simulink model "BPSK_Modem_v1_BMT_012314"  (R2013a)
settings: Solver=ode3  SolverMode=SingleTasking  StartTime=0.0  StopTime=10e3/2400  FixedStep=1/480e3  RelTol=1e-3
values from neighbouring files (symbols this model uses):
  Ki = 2.55    [Costas_Loop_Control_Design.m]
  Ko = ((r*s)/2)^2*H0^2    (= 0.015625)    [Costas_Loop_Control_Design.m]
  Kp = 4.41    [Costas_Loop_Control_Design.m]
  Kv = 2*pi*100    (= 628.318530718)    [Costas_Loop_Control_Design.m]
undefined symbols (not defined in the file or in its folder): DiscIntNeverNeededParam
libraries: commsynccomp2 x3, simulink x3, dspsigops x3, commutil2 x1, commchan3 x1, commrandsrc2 x1, commsink2 x1
settings Model: Creator=tibbs2010  LastModifiedBy=tibbs2010
settings DataIOCC: SignalLoggingSaveFormat=ModelDataLogs
settings DebuggingCC: MultiTaskDSMMsg=warning  MultiTaskCondExecSysMsg=none  StrictBusMsg=None
settings RTWCC: IncludeERTFirstTime=on

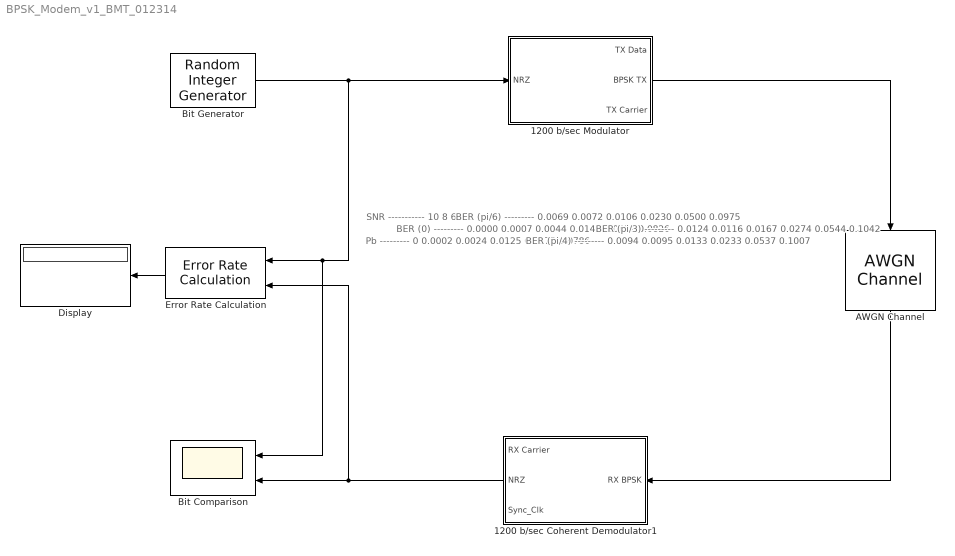
== system BPSK_Modem_v1_BMT_012314 ==
  note: BER (0)
      | ---------
      | 0.0000
      | 0.0007
      | 0.0044
      | 0.0144
      | 0.0432
      | 0.0826
  note: SNR
      | -----------
      |    10
      |      8
      |      6
      |      4
      |      2
      |      0
  note: Pb
      | ---------
      | 0
      | 0.0002
      | 0.0024
      | 0.0125
      | 0.0375
      | 0.0786
  note: BER (pi/6)
      | ---------
      | 0.0069
      | 0.0072
      | 0.0106
      | 0.0230
      | 0.0500
      | 0.0975
  note: BER (pi/4)
      | ---------
      | 0.0094
      | 0.0095
      | 0.0133
      | 0.0233
      | 0.0537
      | 0.1007
  note: BER (pi/3)
      | ---------
      | 0.0124
      | 0.0116
      | 0.0167
      | 0.0274
      | 0.0544
      | 0.1042
  1200 b/sec Modulator : Subsystem
  1200 b/sec Coherent Demodulator1 : Subsystem
  AWGN Channel : commchan3/AWGN Channel  InputProcessing=Columns as channels (frame based)  seed=randseed  noiseMode="Signal to noise ratio  (Eb/No)"  EbNodB=0  EsNodB=10  SNRdB=10  bitsPerSym=1  Ps=12.5  Tsym=1/2400  variance=1
  Bit Comparison : Scope  NumInputPorts=2
      settings: TimeRange=0.008608695652173926  YMin=-0.5~-0.5  YMax=1.5~1.5
  Bit Generator : commrandsrc2/Random Integer Generator  mul=2  seed=randseed  Ts=1/2400  frameBased=off  sampPerFrame=1  orient=off  outDataType=double
  Display : Display
  Error Rate Calculation : commsink2/Error Rate Calculation  N=3  st_delay=0  cp_mode=Entire frame  subframe=[]  PMode=Port  WsName=grayBER  RsMode2=off  stop=off  numErr=1072  maxBits=10e3
  wires:
  Error Rate Calculation/1 -> Display/1
  AWGN Channel/1 -> 1200 b/sec Coherent Demodulator1/1(RX BPSK)
  1200 b/sec Coherent Demodulator1/2(NRZ) -> Error Rate Calculation/2, Bit Comparison/2
  1200 b/sec Modulator/2(BPSK TX) -> AWGN Channel/1
  Bit Generator/1 -> Bit Comparison/1, Error Rate Calculation/1, 1200 b/sec Modulator/1(NRZ)

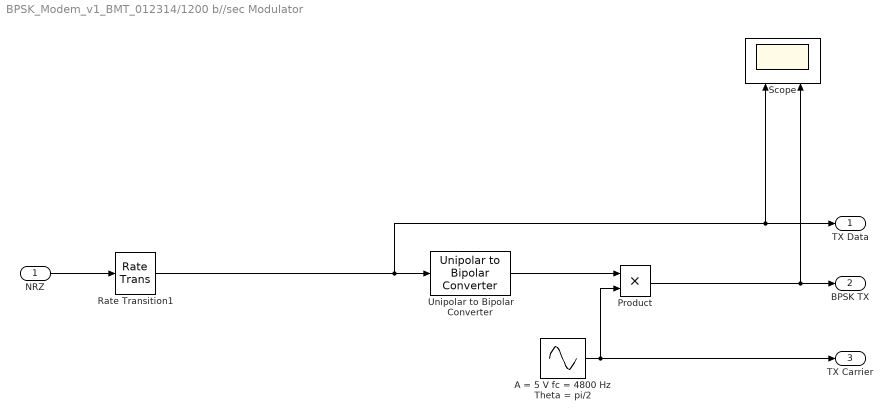
== system BPSK_Modem_v1_BMT_012314/1200 b//sec Modulator ==
  NRZ : Inport
  A = 5 V fc = 4800 Hz Theta = pi/2 : Sin  Amplitude=5  Frequency=2*pi*4800  Phase=pi/2  SampleTime=1/480e3
  Product : Product
  Rate Transition1 : RateTransition  OutPortSampleTime=1/480e3
  Scope : Scope  NumInputPorts=2
      settings: TimeRange=0.06  YMin=-0.5~-0.5  YMax=1.5~1.5  SaveName=ScopeData2
  Unipolar to Bipolar Converter : commutil2/Unipolar to Bipolar Converter  M=2  polarity=Positive  dataType=Inherit via internal rule
  TX Data : Outport
  BPSK TX : Outport  Port=2
  TX Carrier : Outport  Port=3
  wires:
  Rate Transition1/1 -> TX Data/1, Scope/1, Unipolar to Bipolar Converter/1
  Unipolar to Bipolar Converter/1 -> Product/1
  A = 5 V fc = 4800 Hz Theta = pi/2/1 -> TX Carrier/1, Product/2
  NRZ/1 -> Rate Transition1/1
  Product/1 -> Scope/2, BPSK TX/1

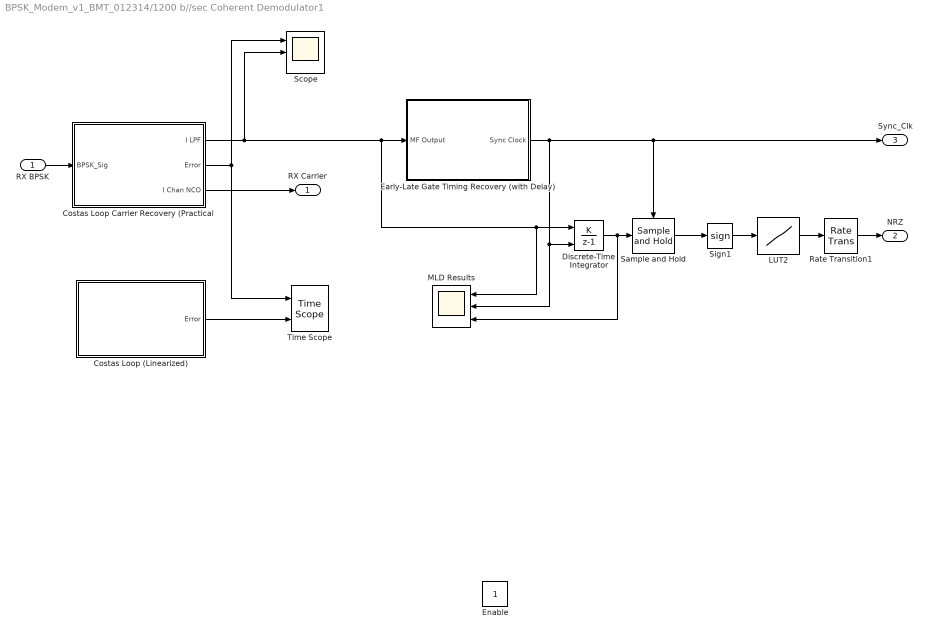
== system BPSK_Modem_v1_BMT_012314/1200 b//sec Coherent Demodulator1 ==
  RX BPSK : Inport
  Costas Loop Carrier Recovery (Practical : Subsystem
  Costas Loop (Linearized) : Subsystem
  Discrete-Time Integrator : DiscreteIntegrator  IntegratorMethod=Accumulation: Forward Euler  ExternalReset=rising  SampleTime=1/480e3  ICPrevOutput=DiscIntNeverNeededParam  ICPrevScaledInput=DiscIntNeverNeededParam
  Early-Late Gate Timing Recovery (with Delay) : Subsystem
  Enable : Constant
  LUT2 : Lookup_n-D  NumberOfTableDimensions=1  BreakpointsForDimension1=[-1 0 1]  Table=[0 0 1]  RndMeth=Simplest  InputSameDT=on
  MLD Results : Scope  NumInputPorts=3
      settings: TimeRange=0.01093750000000002  YMin=-0.5~-0.5~-5  YMax=1.5~1.5~5  SaveName=ScopeData4
  Rate Transition1 : RateTransition  OutPortSampleTime=1/4800
  Sample and Hold : dspsigops/Sample and Hold  trig=Rising edge  initCond=0  latchinput=on
  Scope : Scope  NumInputPorts=3
      settings: TimeRange=0.2  YMin=-0.125~-0.225~-0.5  YMax=0.1~0.225~1.5
  Sign1 : Signum
  Time Scope : TimeScope  NumInputPorts=2  DefaultConfigurationName=spbscopes.TimeScopeBlockCfg
      settings: CopyFcn=scopeextensions.ScopeBlock.callback(gcbh, 'onBlockCopy', gcbh);  DeleteFcn=scopeextensions.ScopeBlock.callback(gcbh, 'onBlockDelete');  PreSaveFcn=scopeextensions.ScopeBlock.callback(gcbh, 'onModelSave');  NameChangeFcn=scopeextensions.ScopeBlock.callback(gcbh, 'onBlockRename');  CloseFcn=scopeextensions.ScopeBlock.callback(gcbh, 'onBlockClose');  PreDeleteFcn=scopeextensions.ScopeBlock.callback(gcbh, 'onBlockPreDelete');
  RX Carrier : Outport
  NRZ : Outport  Port=2
  Sync_Clk : Outport  Port=3
  wires:
  RX BPSK/1 -> Costas Loop Carrier Recovery (Practical/1(BPSK_Sig)
  Sign1/1 -> LUT2/1
  Sample and Hold/1 -> Sign1/1
  LUT2/1 -> Rate Transition1/1
  Costas Loop Carrier Recovery (Practical/2(Error) -> Scope/1, Time Scope/1
  Costas Loop Carrier Recovery (Practical/3(I Chan NCO) -> RX Carrier/1
  Discrete-Time Integrator/1 -> MLD Results/3, Sample and Hold/1
  Rate Transition1/1 -> NRZ/1
  Costas Loop Carrier Recovery (Practical/1(I LPF) -> Scope/2, Early-Late Gate Timing Recovery (with Delay)/1(MF Output), MLD Results/1, Discrete-Time Integrator/1
  Costas Loop (Linearized)/1("Error ") -> Time Scope/2
  Early-Late Gate Timing Recovery (with Delay)/1(Sync Clock) -> Sync_Clk/1, Sample and Hold/Trigger, Discrete-Time Integrator/2, MLD Results/2

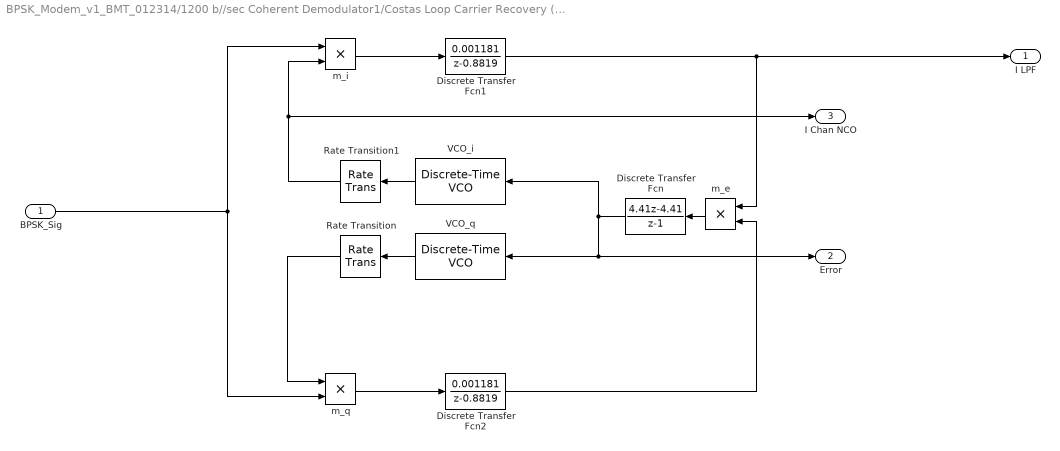
== system BPSK_Modem_v1_BMT_012314/1200 b//sec Coherent Demodulator1/Costas Loop Carrier Recovery (Practical ==
  BPSK_Sig : Inport
  Discrete Transfer Fcn : DiscreteTransferFcn  Numerator=[4.41 -4.41]  Denominator=[1 -1]  SampleTime=1/480e3
  Discrete Transfer Fcn1 : DiscreteTransferFcn  Numerator=[0.001181]  Denominator=[1 -0.8819]  SampleTime=1/480e3
  Discrete Transfer Fcn2 : DiscreteTransferFcn  Numerator=[0.001181]  Denominator=[1 -0.8819]  SampleTime=1/480e3
  Rate Transition : RateTransition  OutPortSampleTime=1/480e3
  Rate Transition1 : RateTransition  OutPortSampleTime=1/480e3
  VCO_i : commsynccomp2/Discrete-Time VCO  Ac=5  Fc=4800  Kc=100  Ph=pi/6  ts=1/480e3
  VCO_q : commsynccomp2/Discrete-Time VCO  Ac=5  Fc=4800  Kc=100  Ph=pi/2+pi/6  ts=1/480e3
  m_e : Product  SampleTime=1/480e3
  m_i : Product  SampleTime=1/480e3
  m_q : Product  SampleTime=1/480e3
  I LPF : Outport
  Error : Outport  Port=2
  I Chan NCO : Outport  Port=3
  wires:
  VCO_i/1 -> Rate Transition1/1
  VCO_q/1 -> Rate Transition/1
  Rate Transition/1 -> m_q/1
  Rate Transition1/1 -> m_i/2, I Chan NCO/1
  m_q/1 -> Discrete Transfer Fcn2/1
  m_i/1 -> Discrete Transfer Fcn1/1
  BPSK_Sig/1 -> m_i/1, m_q/2
  m_e/1 -> Discrete Transfer Fcn/1
  Discrete Transfer Fcn2/1 -> m_e/2
  Discrete Transfer Fcn/1 -> VCO_i/1, Error/1, VCO_q/1
  Discrete Transfer Fcn1/1 -> I LPF/1, m_e/1

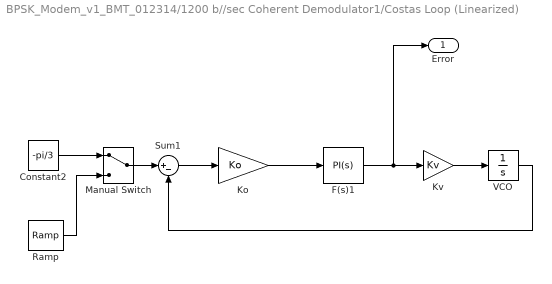
== system BPSK_Modem_v1_BMT_012314/1200 b//sec Coherent Demodulator1/Costas Loop (Linearized) ==
  Constant2 : Constant  Value=-pi/3
  F(s)1 : simulink/Continuous/PID Controller  Controller=PI  TimeDomain=Continuous-time  SampleTime=1/480e3  IntegratorMethod=Forward Euler  FilterMethod=Forward Euler  Form=Parallel  P=Kp  I=Ki  D=0  N=1  InitialConditionSource=internal  InitialConditionForIntegrator=0  InitialConditionForFilter=0  ExternalReset=none  LimitOutput=off  UpperSaturationLimit=inf  LowerSaturationLimit=-inf  LinearizeAsGain=on  AntiWindupMode=none  Kb=1  TrackingMode=off  Kt=1  PParamMin=[]  PParamMax=[]  IParamMin=[]  IParamMax=[]  DParamMin=[]  DParamMax=[]  NParamMin=[]  NParamMax=[]  KbParamMin=[]  KbParamMax=[]  KtParamMin=[]  KtParamMax=[]  POutMin=[]  POutMax=[]  IOutMin=[]  IOutMax=[]  DOutMin=[]  DOutMax=[]  NOutMin=[]  NOutMax=[]  KbOutMin=[]  KbOutMax=[]  KtOutMin=[]  KtOutMax=[]  IntegratorOutMin=[]  IntegratorOutMax=[]  FilterOutMin=[]  FilterOutMax=[]  SumOutMin=[]  SumOutMax=[]  SumI1OutMin=[]  SumI1OutMax=[]  SumI2OutMin=[]  SumI2OutMax=[]  SumI3OutMin=[]  SumI3OutMax=[]  SumDOutMin=[]  SumDOutMax=[]  SaturationOutMin=[]  SaturationOutMax=[]  IntegratorContinuousStateAttributes=''  IntegratorStateMustResolveToSignalObject=off  IntegratorRTWStateStorageClass=Auto  FilterContinuousStateAttributes=''  FilterStateMustResolveToSignalObject=off  FilterRTWStateStorageClass=Auto
  Ko : Gain  Gain=Ko
  Kv : Gain  Gain=Kv
  Manual Switch : ManualSwitch
  Ramp : simulink/Sources/Ramp  slope=-2*pi*3  start=0  X0=0
  Sum1 : Sum  Inputs=|+-
  VCO : Integrator
  "Error " : Outport
  wires:
  F(s)1/1 -> "Error "/1, Kv/1
  VCO/1 -> Sum1/2
  Kv/1 -> VCO/1
  Ko/1 -> F(s)1/1
  Sum1/1 -> Ko/1
  Manual Switch/1 -> Sum1/1
  Constant2/1 -> Manual Switch/1
  Ramp/1 -> Manual Switch/2

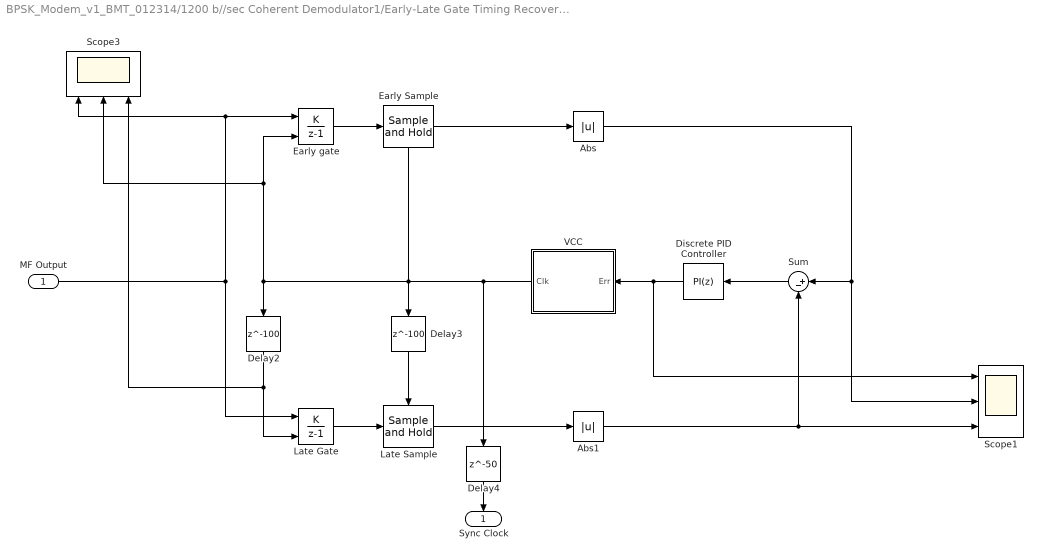
== system BPSK_Modem_v1_BMT_012314/1200 b//sec Coherent Demodulator1/Early-Late Gate Timing Recovery (with Delay) ==
  MF Output : Inport
  Abs : Abs
  Abs1 : Abs
  Delay2 : Delay  DelayLength=100  InitialCondition=0
  Delay3 : Delay  DelayLength=100  InitialCondition=0
  Delay4 : Delay  DelayLength=50  InitialCondition=0
  Discrete PID Controller : simulink/Continuous/PID Controller  Controller=PI  TimeDomain=Discrete-time  SampleTime=1/480e3  IntegratorMethod=Forward Euler  FilterMethod=Forward Euler  Form=Parallel  P=0.05  I=0.25  D=0  N=1  InitialConditionSource=internal  InitialConditionForIntegrator=0  InitialConditionForFilter=0  ExternalReset=none  LimitOutput=off  UpperSaturationLimit=inf  LowerSaturationLimit=-inf  LinearizeAsGain=off  AntiWindupMode=none  Kb=1  TrackingMode=off  Kt=1  PParamMin=[]  PParamMax=[]  IParamMin=[]  IParamMax=[]  DParamMin=[]  DParamMax=[]  NParamMin=[]  NParamMax=[]  KbParamMin=[]  KbParamMax=[]  KtParamMin=[]  KtParamMax=[]  POutMin=[]  POutMax=[]  IOutMin=[]  IOutMax=[]  DOutMin=[]  DOutMax=[]  NOutMin=[]  NOutMax=[]  KbOutMin=[]  KbOutMax=[]  KtOutMin=[]  KtOutMax=[]  IntegratorOutMin=[]  IntegratorOutMax=[]  FilterOutMin=[]  FilterOutMax=[]  SumOutMin=[]  SumOutMax=[]  SumI1OutMin=[]  SumI1OutMax=[]  SumI2OutMin=[]  SumI2OutMax=[]  SumI3OutMin=[]  SumI3OutMax=[]  SumDOutMin=[]  SumDOutMax=[]  SaturationOutMin=[]  SaturationOutMax=[]  IntegratorContinuousStateAttributes=''  IntegratorStateMustResolveToSignalObject=off  IntegratorRTWStateStorageClass=Auto  FilterContinuousStateAttributes=''  FilterStateMustResolveToSignalObject=off  FilterRTWStateStorageClass=Auto
  Early Sample : dspsigops/Sample and Hold  trig=Rising edge  initCond=0  latchinput=on
  Early gate : DiscreteIntegrator  IntegratorMethod=Accumulation: Forward Euler  gainval=1  ExternalReset=rising  SampleTime=1/480e3  ICPrevOutput=DiscIntNeverNeededParam  ICPrevScaledInput=DiscIntNeverNeededParam
  Late Gate : DiscreteIntegrator  IntegratorMethod=Accumulation: Forward Euler  gainval=1  ExternalReset=rising  SampleTime=1/480e3  ICPrevOutput=DiscIntNeverNeededParam  ICPrevScaledInput=DiscIntNeverNeededParam
  Late Sample : dspsigops/Sample and Hold  trig=Rising edge  initCond=0  latchinput=on
  Scope1 : Scope  NumInputPorts=3
      settings: TimeRange=0.06  YMin=-0.7~0~0  YMax=0.9~9~18  SaveName=ScopeData5
  Scope3 : Scope  NumInputPorts=3
      settings: TimeRange=0.06  YMin=-0.5~-0.5~-0.5  YMax=1.5~1.5~1.5  SaveName=ScopeData7
  Sum : Sum  Inputs=|+-
  VCC : Subsystem
  Sync Clock : Outport
  wires:
  Late Sample/1 -> Abs1/1
  Sum/1 -> Discrete PID Controller/1
  Early gate/1 -> Early Sample/1
  Late Gate/1 -> Late Sample/1
  Discrete PID Controller/1 -> Scope1/1, VCC/1(Err)
  Early Sample/1 -> Abs/1
  Delay3/1 -> Late Sample/Trigger
  Delay2/1 -> Scope3/3, Late Gate/2
  VCC/1(Clk) -> Delay4/1, Delay3/1, Early Sample/Trigger, Scope3/2, Early gate/2, Delay2/1
  MF Output/1 -> Early gate/1, Scope3/1, Late Gate/1
  Delay4/1 -> Sync Clock/1
  Abs1/1 -> Sum/2, Scope1/3
  Abs/1 -> Scope1/2, Sum/1

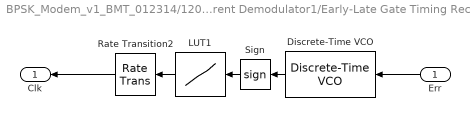
== system BPSK_Modem_v1_BMT_012314/1200 b//sec Coherent Demodulator1/Early-Late Gate Timing Recovery (with Delay)/VCC ==
  Err : Inport
  Discrete-Time VCO : commsynccomp2/Discrete-Time VCO  Ac=1  Fc=2400  Kc=3  Ph=pi/6  ts=1/480e3
  LUT1 : Lookup_n-D  NumberOfTableDimensions=1  BreakpointsForDimension1=[-1 0 1]  Table=[0 0 1]  RndMeth=Simplest  InputSameDT=on
  Rate Transition2 : RateTransition  OutPortSampleTime=1/480e3
  Sign : Signum
  Clk : Outport
  wires:
  Discrete-Time VCO/1 -> Sign/1
  Err/1 -> Discrete-Time VCO/1
  LUT1/1 -> Rate Transition2/1
  Rate Transition2/1 -> Clk/1
  Sign/1 -> LUT1/1
